simulink model "tanque_opcional_caudal_var"  (R2020b)
settings: Solver=VariableStepAuto  StartTime=0.0  StopTime=5000  FixedStep=0.1  RelTol=1e-3
settings Model: Creator=Darkhorrow  LastModifiedBy=Darkhorrow

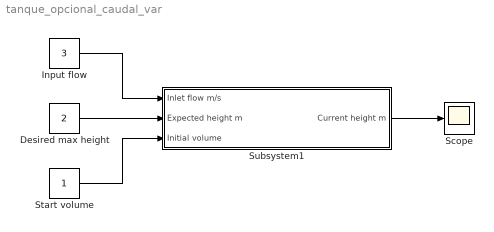
== system tanque_opcional_caudal_var ==
  Desired max height : Constant  Value=2
  Input flow : Constant  Value=3
  Scope : Scope
  Start volume : Constant
  Subsystem1 : Subsystem
  wires:
  Subsystem1/1(Current height m) -> Scope/1
  Input flow/1 -> Subsystem1/1(Inlet flow m/s)
  Desired max height/1 -> Subsystem1/2(Expected height m)
  Start volume/1 -> Subsystem1/3(Initial volume)

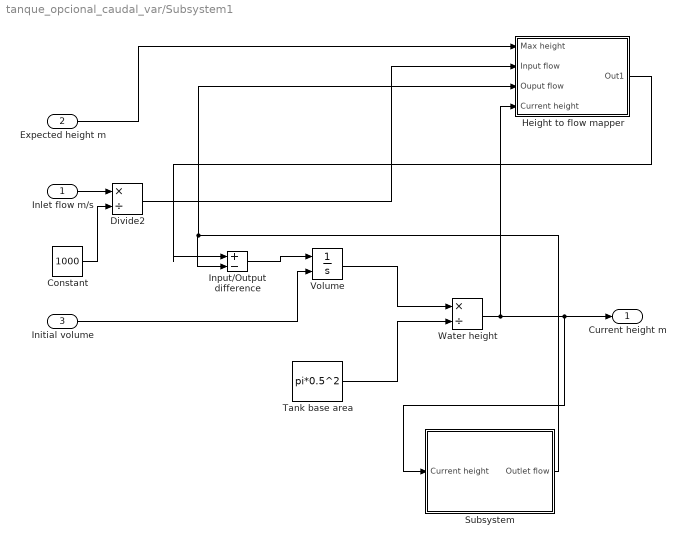
== system tanque_opcional_caudal_var/Subsystem1 ==
  Inlet flow m/s : Inport
  Expected height m : Inport  Port=2
  Initial volume : Inport  Port=3
  Constant : Constant  Value=1000
  Divide2 : Product  Inputs=*/
  Height to flow mapper : Subsystem
  Input/Output difference : Sum  Inputs=|+-
  Subsystem : Subsystem
  Tank base area : Constant  Value=pi*0.5^2
  Volume : Integrator  InitialConditionSource=external
  Water height : Product  Inputs=*/
  Current height m : Outport
  wires:
  Input/Output difference/1 -> Volume/1
  Constant/1 -> Divide2/2
  Subsystem/1("Outlet flow ") -> Height to flow mapper/3(" Ouput flow"), Input/Output difference/2
  Tank base area/1 -> Water height/2
  Height to flow mapper/1(Out1) -> Input/Output difference/1
  Water height/1 -> Current height m/1, Subsystem/1(Current height), Height to flow mapper/4(Current height)
  Initial volume/1 -> Volume/2
  Volume/1 -> Water height/1
  Divide2/1 -> Height to flow mapper/2(Input flow)
  Expected height m/1 -> Height to flow mapper/1(Max height)
  Inlet flow m/s/1 -> Divide2/1

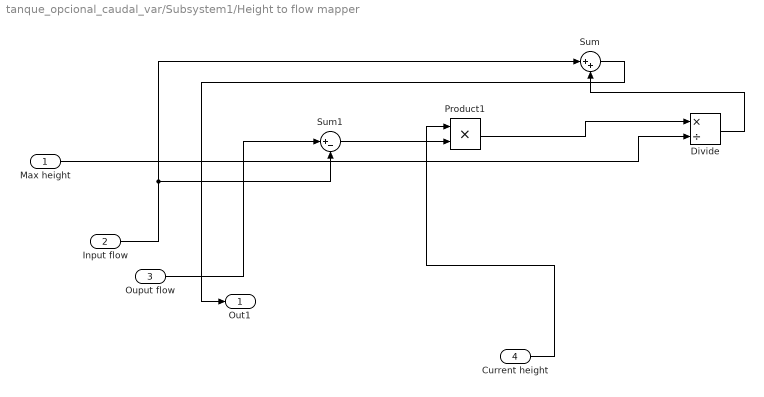
== system tanque_opcional_caudal_var/Subsystem1/Height to flow mapper ==
  Max height : Inport
  Input flow : Inport  Port=2
  " Ouput flow" : Inport  Port=3
  Current height : Inport  Port=4
  Divide : Product  Inputs=*/
  Product1 : Product
  Sum : Sum  Inputs=|++
  Sum1 : Sum  Inputs=|+-
  Out1 : Outport
  wires:
  Sum1/1 -> Product1/2
  Product1/1 -> Divide/1
  Input flow/1 -> Sum/1, Sum1/2
  Divide/1 -> Sum/2
  Current height/1 -> Product1/1
  " Ouput flow"/1 -> Sum1/1
  Sum/1 -> Out1/1
  Max height/1 -> Divide/2

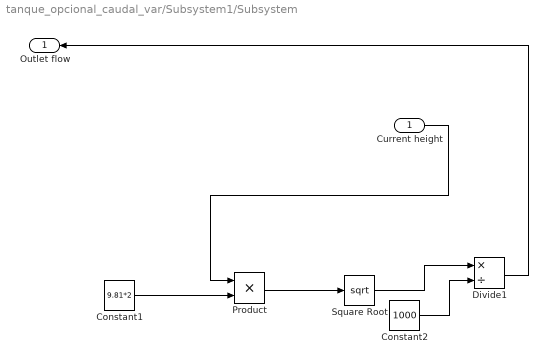
== system tanque_opcional_caudal_var/Subsystem1/Subsystem ==
  Current height : Inport
  Constant1 : Constant  Value=9.81*2
  Constant2 : Constant  Value=1000
  Divide1 : Product  Inputs=*/
  Product : Product
  Square Root : Sqrt  SaturateOnIntegerOverflow=on
  "Outlet flow " : Outport
  wires:
  Product/1 -> Square Root/1
  Constant1/1 -> Product/2
  Constant2/1 -> Divide1/2
  Current height/1 -> Product/1
  Square Root/1 -> Divide1/1
  Divide1/1 -> "Outlet flow "/1
